simulink model "lab5q1_sys"  (R2023b)
settings: Solver=VariableStepAuto  StartTime=0.0  StopTime=10  RelTol=1e-3
libraries: cstblocks x2
settings Model: Creator=piercest  LastModifiedBy=piercest

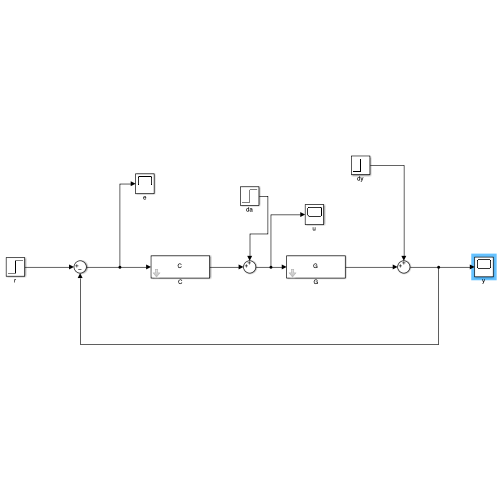
[thumbnail: Simulink's stored preview of the top-level diagram]
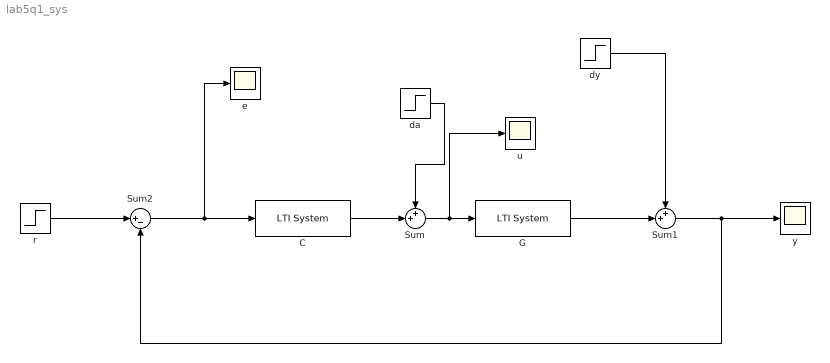
== system lab5q1_sys ==
  C : cstblocks/LTI System  sys=C  IC=[]  PadeOrder=0
  G : cstblocks/LTI System  sys=G  IC=[]  PadeOrder=0
  Sum : Sum  Inputs=++|
  Sum1 : Sum  Inputs=++|
  Sum2 : Sum  Inputs=|+-
  da : Step  Time=0  After=0  SampleTime=0  VectorParams1D=off
  dy : Step  Time=0  After=2  SampleTime=0  VectorParams1D=off
  e : Scope
  r : Step  Time=0  After=3  SampleTime=0
  u : Scope
  y : Scope
  wires:
  C/1 -> Sum/2
  Sum/1 -> u/1, G/1
  da/1 -> Sum/1
  G/1 -> Sum1/2
  r/1 -> Sum2/1
  Sum1/1 -> y/1, Sum2/2
  Sum2/1 -> e/1, C/1
  dy/1 -> Sum1/1
